simulink model "validation"  (Simulink 7.9)
settings: Solver=ode4  StartTime=0.0  StopTime=600  FixedStep=0.1  RelTol=1e-3
libraries: aerolib6dof2 x1
settings Model: Creator=benelgiz  LastModifiedBy=benelgiz

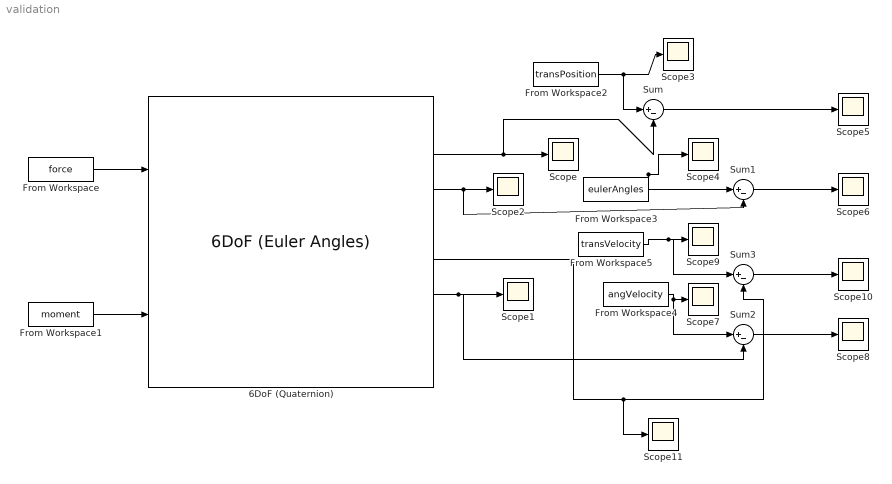
== system validation ==
  6DoF (Quaternion) : aerolib6dof2/6DoF (Euler Angles)  units=Metric (MKS)  mtype=Fixed  rep=Quaternion  xme_0=[0 0 0]  Vm_0=[1e-5 1e-5 1e-5]  eul_0=[0 0 0]  pm_0=[0 0 0]  mass_0=28  mass_e=0  mass_f=0  inertia=[2.56 0 0.5; 0 10.9 0; 0.5 0 11.3]  inertia_e=eye(3)  inertia_f=eye(3)  k_quat=1.0
  From Workspace : FromWorkspace  VariableName=force  SampleTime=0
  From Workspace1 : FromWorkspace  VariableName=moment  SampleTime=0
  From Workspace2 : FromWorkspace  VariableName=transPosition  SampleTime=0
  From Workspace3 : FromWorkspace  VariableName=eulerAngles  SampleTime=0
  From Workspace4 : FromWorkspace  VariableName=angVelocity  SampleTime=0
  From Workspace5 : FromWorkspace  VariableName=transVelocity  SampleTime=0
  Scope{,1..11} (12 alike) : Scope
      Scope10 settings: SaveName=ScopeData9
      Scope11 settings: SaveName=ScopeData11
      Scope2 settings: TimeRange=500  YMin=-4  YMax=4  SaveName=ScopeData2
      Scope3 settings: SaveName=ScopeData3
      Scope4 settings: SaveName=ScopeData4
      Scope5 settings: SaveName=ScopeData5
      Scope6 settings: SaveName=ScopeData6
      Scope7 settings: SaveName=ScopeData7
      Scope8 settings: SaveName=ScopeData8
      Scope9 settings: SaveName=ScopeData10
  Sum{,1..3} (4 alike) : Sum  Inputs=|+-
  wires:
  From Workspace/1 -> 6DoF (Quaternion)/1
  From Workspace1/1 -> 6DoF (Quaternion)/2
  6DoF (Quaternion)/2 -> Scope/1, Sum/2
  6DoF (Quaternion)/6 -> Scope1/1, Sum2/2
  6DoF (Quaternion)/3 -> Scope2/1, Sum1/2
  From Workspace2/1 -> Sum/1, Scope3/1
  From Workspace3/1 -> Scope4/1, Sum1/1
  Sum/1 -> Scope5/1
  Sum1/1 -> Scope6/1
  Sum2/1 -> Scope8/1
  From Workspace4/1 -> Sum2/1, Scope7/1
  Sum3/1 -> Scope10/1
  From Workspace5/1 -> Sum3/1, Scope9/1
  6DoF (Quaternion)/5 -> Sum3/2, Scope11/1
